simulink model "StateSpaceController_Observability"  (R2021a)
settings: Solver=FixedStepAuto  StartTime=0.0  StopTime=SimTime-Ts  FixedStep=1e-3  RelTol=1e-3
values from neighbouring files (symbols this model uses):
  a0 = A_q(3)    [PIDModalController.m]    (also in PolynomialController.m)
  a1 = A_q(2)    [PIDModalController.m]    (also in PolynomialController.m)
  a2 = A_q(1)    [PIDModalController.m]    (also in PolynomialController.m)
  b0 = B_q(1)    [PIDModalController.m]    (also in PolynomialController.m)
  C12 = x(3)    [DigitalPIDRunner.m]    (also in DoubleMassRunner.m; NNIdentify.m = Xnt_noise(3); NNTrainingSet.m = T(i, 3); PIDModalController.m = 16.6338)
  k1 = x(1)    [DigitalPIDRunner.m]    (also in DoubleMassRunner.m; NNIdentify.m = Xnt_noise(1); NNTrainingSet.m = T(i, 1); PIDModalController.m = 0.2244)
  k2 = x(2)    [DigitalPIDRunner.m]    (also in DoubleMassRunner.m; NNIdentify.m = Xnt_noise(2); NNTrainingSet.m = T(i, 2); PIDModalController.m = 0.5636)
  Ts = 1e-3    (= 0.001)    [DigitalPIDRunner.m]    (also in DoubleMassRunner.m = ref.Ts; NNTrainingSet.m; PIDModalController.m; PIDRunner.m = p.Results.StepTime)
undefined symbols (not defined in the file or in its folder): b1, dss0, K_canobs, L_obs
settings Model: Creator=akangmufti  LastModifiedBy=akangmufti

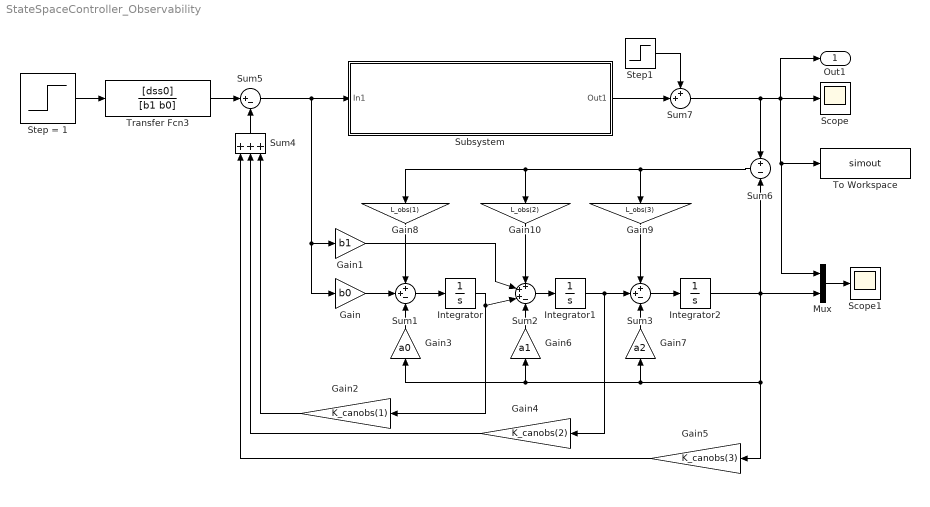
== system StateSpaceController_Observability ==
  Gain : Gain  Gain=b0
  Gain1 : Gain  Gain=b1
  Gain10 : Gain  Gain=L_obs(2)
  Gain2 : Gain  Gain=K_canobs(1)
  Gain3 : Gain  Gain=a0
  Gain4 : Gain  Gain=K_canobs(2)
  Gain5 : Gain  Gain=K_canobs(3)
  Gain6 : Gain  Gain=a1
  Gain7 : Gain  Gain=a2
  Gain8 : Gain  Gain=L_obs(1)
  Gain9 : Gain  Gain=L_obs(3)
  Integrator : Integrator
  Integrator1 : Integrator
  Integrator2 : Integrator
  Mux : Mux  Inputs=2
  Scope : Scope
  Scope1 : Scope
  Step = 1 : Step  Time=0.0001  SampleTime=0
  Step1 : Step  Time=2  After=-0.5  SampleTime=0
  Subsystem : Subsystem
  Sum1 : Sum  Inputs=++-
  Sum2 : Sum  Inputs=+++-
  Sum3 : Sum  Inputs=++-
  Sum4 : Sum  Inputs=+++
  Sum5 : Sum  Inputs=|+-
  Sum6 : Sum  Inputs=+|-
  Sum7 : Sum  Inputs=++|
  To Workspace : ToWorkspace  VariableName=simout  SampleTime=Ts
      settings: Save2DSignal=2-D array (concatenate along first dimension)
  Transfer Fcn3 : TransferFcn  Numerator=[dss0]  Denominator=[b1 b0]  ContinuousStateAttributes='x1'
  Out1 : Outport
  wires:
  Gain2/1 -> Sum4/3
  Gain4/1 -> Sum4/2
  Gain5/1 -> Sum4/1
  Sum4/1 -> Sum5/2
  Sum7/1 -> Sum6/1, Mux/1, To Workspace/1, Out1/1, Scope/1
  Sum5/1 -> Subsystem/1(In1), Gain/1, Gain1/1
  Sum1/1 -> Integrator/1
  Integrator1/1 -> Sum3/2, Gain4/1
  Integrator/1 -> Gain2/1, Sum2/3
  Integrator2/1 -> Gain3/1, Gain6/1, Gain7/1, Gain5/1, Mux/2, Sum6/2
  Mux/1 -> Scope1/1
  Transfer Fcn3/1 -> Sum5/1
  Step = 1/1 -> Transfer Fcn3/1
  Subsystem/1(Out1) -> Sum7/2
  Step1/1 -> Sum7/1
  Gain3/1 -> Sum1/3
  Gain/1 -> Sum1/2
  Gain8/1 -> Sum1/1
  Gain1/1 -> Sum2/2
  Gain10/1 -> Sum2/1
  Gain6/1 -> Sum2/4
  Sum2/1 -> Integrator1/1
  Gain9/1 -> Sum3/1
  Sum3/1 -> Integrator2/1
  Gain7/1 -> Sum3/3
  Sum6/1 -> Gain8/1, Gain10/1, Gain9/1

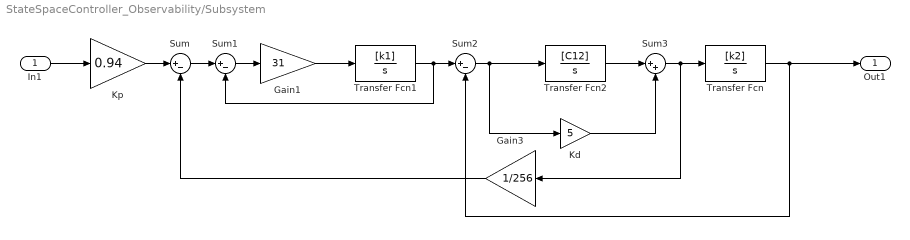
== system StateSpaceController_Observability/Subsystem ==
  In1 : Inport
  Gain1 : Gain  Gain=31
  Gain3 : Gain  Gain=1/256
  Kd : Gain  Gain=5
  Kp : Gain  Gain=0.94
  Sum : Sum  Inputs=|+-
  Sum1 : Sum  Inputs=|+-
  Sum2 : Sum  Inputs=|+-
  Sum3 : Sum  Inputs=|++
  Transfer Fcn : TransferFcn  Numerator=[k2]  Denominator=[1 0]  ContinuousStateAttributes='x3'
  Transfer Fcn1 : TransferFcn  Numerator=[k1]  Denominator=[1 0]  ContinuousStateAttributes='x1'
  Transfer Fcn2 : TransferFcn  Numerator=[C12]  Denominator=[1 0]  ContinuousStateAttributes='x2'
  Out1 : Outport
  wires:
  Gain1/1 -> Transfer Fcn1/1
  Kd/1 -> Sum3/2
  Sum2/1 -> Kd/1, Transfer Fcn2/1
  Sum3/1 -> Gain3/1, Transfer Fcn/1
  Transfer Fcn2/1 -> Sum3/1
  Sum1/1 -> Gain1/1
  Transfer Fcn1/1 -> Sum1/2, Sum2/1
  Transfer Fcn/1 -> Out1/1, Sum2/2
  Sum/1 -> Sum1/1
  Kp/1 -> Sum/1
  Gain3/1 -> Sum/2
  In1/1 -> Kp/1
